simulink model "MRD_FDFV"  (R2021b)
settings: Solver=FixedStepAuto  StartTime=0.0  StopTime=1  FixedStep=1e-4  RelTol=1e-3
InitFcn:
  | clear ; clc
  | SimTime = 6;                   % Simulation Time
  | Gn0=16e-6;
  | v=10;
  | Volt = 0;
  | Vmax = 2;
  | fz = 10;
  | wc = 2*pi*fz;
  | 
  | 
  | 
  | 
  | c0a=784;
  | c0b=1803;
  | k0=3610;
  | c1a=14649;
  | c1b=34622;
  | k1=840;
  | x0=0.0245;
  | alph_a=12441;
  | alph_b=38430;
  | gamma=136320;
  | bta=2059020;
  | A=58;
  | n=2;
  | eta=190;
  | 
  | c0_a=784;
  | c0_b=1803;
  | k0=3610;
  | c1_a=14649;
  | c1_b=34622;
  | k1=840;
  | x0=0.0245;
  | alpha_a=12441;
  | alpha_b=38430;
  | gamma=136320;
  | A=58;
  | beta=2059020;
  | eta=190;              % Not available in the above parameters
  | n=2;
settings Model: Creator=Yoga  LastModifiedBy=baig
settings DebuggingCC: UnconnectedInputMsg=none  UnconnectedOutputMsg=none  UnconnectedLineMsg=none
settings RTWCC: GPUComputeCapability=5.0  DLArmComputeVersion=20.02.1
settings ConfigComp: CovBoundaryAbsTol=1.0e-5

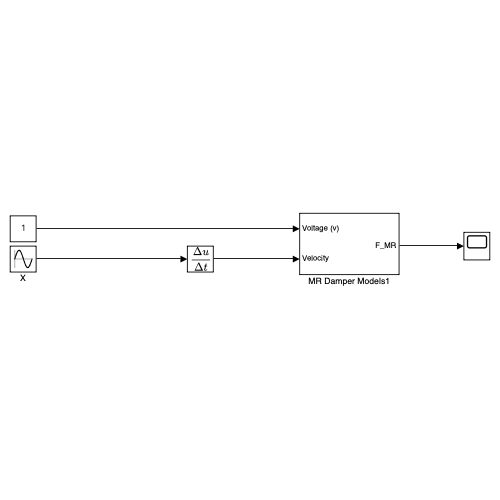
[thumbnail: Simulink's stored preview of the top-level diagram]
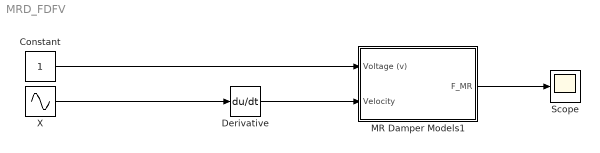
== system MRD_FDFV ==
  Constant : Constant
  Derivative : Derivative
  MR Damper Models1 : Subsystem
  Scope : Scope
  X : Sin  Amplitude=0.008  Frequency=2*pi*10  Phase=-pi/2  SampleTime=0
  wires:
  Constant/1 -> MR Damper Models1/1(Voltage (v))
  MR Damper Models1/1(F_MR) -> Scope/1
  X/1 -> Derivative/1
  Derivative/1 -> MR Damper Models1/2(Velocity)

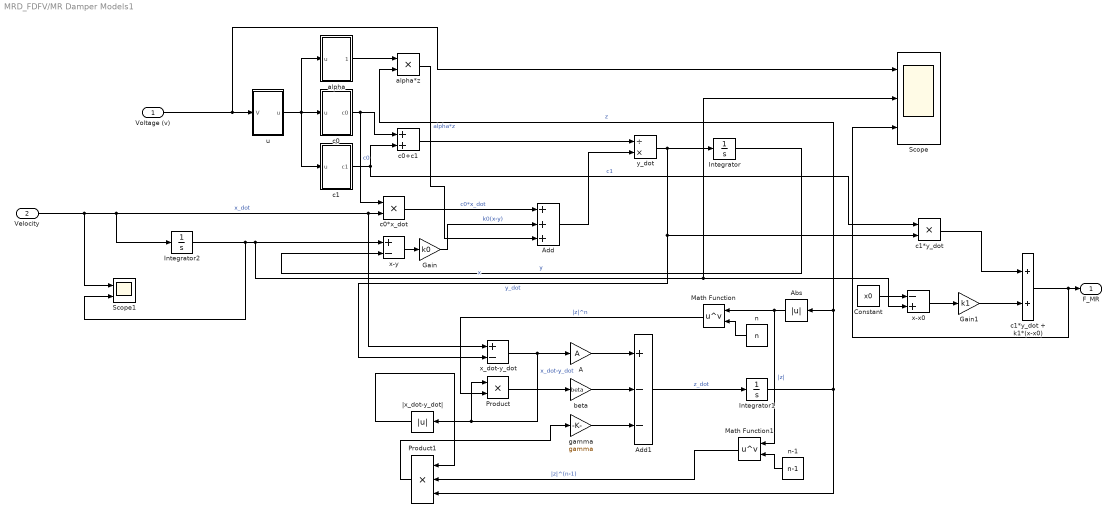
== system MRD_FDFV/MR Damper Models1 ==
  Voltage (v) : Inport
  Velocity : Inport  Port=2
  A : Gain  Gain=A
  Abs : Abs
  Add : Sum  Inputs=+++
  Add1 : Sum  Inputs=+--
  Constant : Constant  Value=x0
  Gain : Gain  Gain=k0
  Gain1 : Gain  Gain=k1
  Integrator : Integrator
  Integrator1 : Integrator  UpperSaturationLimit=0.01  LowerSaturationLimit=0
  Integrator2 : Integrator
  Math Function : Math  Operator=pow  SignedPower=on  SaturateOnIntegerOverflow=on
  Math Function1 : Math  Operator=pow  SignedPower=on  SaturateOnIntegerOverflow=on
  Product : Product
  Product1 : Product  Inputs=3
  Scope : Scope  NumInputPorts=3
  Scope1 : Scope  NumInputPorts=2
  alpha : Subsystem
  alpha*z : Product
  beta : Gain  Gain=beta
  c0 : Subsystem
  c0*x_dot : Product
  c0+c1 : Sum
  c1 : Subsystem
  c1*y_dot : Product
  c1*y_dot + k1*(x-x0) : Sum
  gamma : Gain  Gain=gamma
  n : Constant  Value=n
  n-1 : Constant  Value=n-1
  u : Subsystem
  x-x0 : Sum  Inputs=-+
  x-y : Sum  Inputs=+-
  x_dot-y_dot : Sum  Inputs=+-
  y_dot : Product  Inputs=/*
  |x_dot-y_dot| : Abs
  F_MR : Outport
  wires:
  Abs/1 -> Math Function/1, Math Function1/1  "|z|"
  Constant/1 -> x-x0/1
  Math Function/1 -> Product/2  "|z|^n"
  Product/1 -> beta/1
  n/1 -> Math Function/2
  Integrator1/1 -> Product1/3, Abs/1, alpha*z/2  "z"
  x-x0/1 -> Gain1/1
  x_dot-y_dot/1 -> A/1, Product/1, |x_dot-y_dot|/1  "x_dot-y_dot"
  A/1 -> Add1/1
  Add1/1 -> Integrator1/1  "z_dot"
  Integrator/1 -> x-y/2  "y"
  y_dot/1 -> Integrator/1, x_dot-y_dot/2, c1*y_dot/2  "y_dot"
  Product1/1 -> gamma/1
  Math Function1/1 -> Product1/2  "|z|^(n-1)"
  n-1/1 -> Math Function1/2
  c0/1(c0) -> c0+c1/1, c0*x_dot/1  "c0"
  c1/1(c1) -> c1*y_dot/1, c0+c1/2  "c1"
  u/1(u) -> alpha/1(u), c1/1(u), c0/1(u)
  Gain/1 -> Add/2  "k0(x-y)"
  c0*x_dot/1 -> Add/1  "c0*x_dot"
  Gain1/1 -> c1*y_dot + k1*(x-x0)/2
  c1*y_dot/1 -> c1*y_dot + k1*(x-x0)/1
  alpha*z/1 -> Add/3  "alpha*z"
  alpha/1(alpha) -> alpha*z/1
  x-y/1 -> Gain/1
  Velocity/1 -> c0*x_dot/2, x_dot-y_dot/1, Integrator2/1, Scope1/1  "x_dot"
  |x_dot-y_dot|/1 -> Product1/1
  Add/1 -> y_dot/2
  gamma/1 -> Add1/3
  beta/1 -> Add1/2
  c0+c1/1 -> y_dot/1
  Voltage (v)/1 -> Scope/1, u/1(V)
  c1*y_dot + k1*(x-x0)/1 -> Scope/3, F_MR/1
  Integrator2/1 -> Scope1/2, Scope/2, x-x0/2, x-y/1  "x"

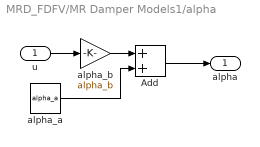
== system MRD_FDFV/MR Damper Models1/alpha ==
  u : Inport
  Add : Sum
  alpha_a : Constant  Value=alpha_a
  alpha_b : Gain  Gain=alpha_b
  alpha : Outport
  wires:
  Add/1 -> alpha/1
  alpha_a/1 -> Add/2
  u/1 -> alpha_b/1
  alpha_b/1 -> Add/1

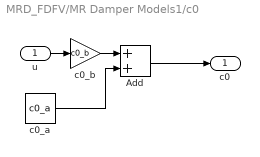
== system MRD_FDFV/MR Damper Models1/c0 ==
  u : Inport
  Add : Sum
  c0_a : Constant  Value=c0_a
  c0_b : Gain  Gain=c0_b
  c0 : Outport
  wires:
  Add/1 -> c0/1
  c0_a/1 -> Add/2
  u/1 -> c0_b/1
  c0_b/1 -> Add/1

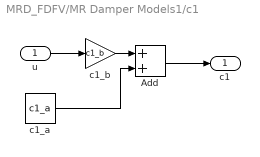
== system MRD_FDFV/MR Damper Models1/c1 ==
  u : Inport
  Add : Sum
  c1_a : Constant  Value=c1_a
  c1_b : Gain  Gain=c1_b
  c1 : Outport
  wires:
  Add/1 -> c1/1
  c1_a/1 -> Add/2
  u/1 -> c1_b/1
  c1_b/1 -> Add/1

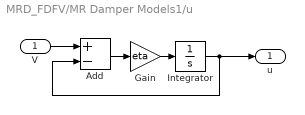
== system MRD_FDFV/MR Damper Models1/u ==
  V : Inport
  Add : Sum  Inputs=+-
  Gain : Gain  Gain=eta
  Integrator : Integrator
  u : Outport
  wires:
  Integrator/1 -> Add/2, u/1
  Gain/1 -> Integrator/1
  Add/1 -> Gain/1
  V/1 -> Add/1
